simulink model "vision_try3_work"  (R2016b)
settings: Solver=VariableStepAuto  StartTime=0.0  StopTime=inf  RelTol=1e-3
undefined symbols (not defined in the file): gray
libraries: dspvision x1, visionsources x1, visionanalysis x1
settings Model: Creator=bhawnath.tiwari  LastModifiedBy=bhawnath.tiwari

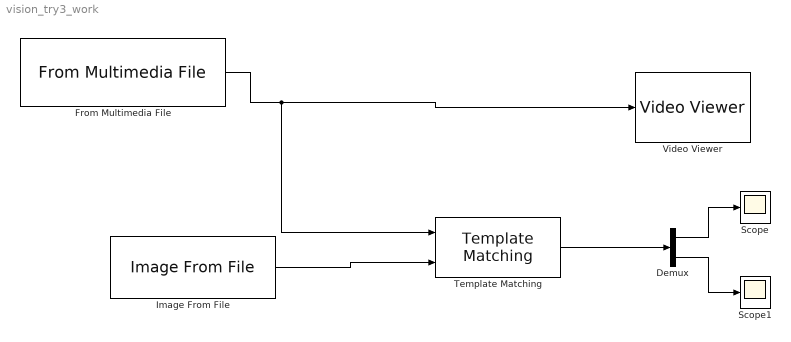
== system vision_try3_work ==
  Demux : Demux  Outputs=2
  From Multimedia File : dspvision/From Multimedia File  inputFilename=G:\Utilisateurs\bhawnath.tiwari\Documents\MATLAB\testr1.avi  loop=on  numPlays=inf  outputStreams=Video only  videoDataType=double  audioDataType=int16  inheritSampleTime=on  userDefinedSampleTime=1/30  noAudioOutput=off  isIntensityVideo=off  fourcc=Intensity  colorVideoFormat=One multidimensional signal  outputEOF=off  dataOrg=Column-major  audioFrameSize=1024  computeAudioFrameSize=off  outSamplingMode=Sample based
  Image From File : visionsources/Image From File  Tag=vipblks_nd  FileName=G:\Utilisateurs\bhawnath.tiwari\Documents\MATLAB\testr1_bolt.png  imagePorts=One multidimensional signal  Ts=inf  ImageDataType=double  Signed=on  WordLength=16  sdImageDataType=uint(8)  FractionLengthMode=User-defined  FractionLength=15  OutPortLabels=R|G|B
  Scope : Scope
  Scope1 : Scope
  Template Matching : visionanalysis/Template Matching  metric=Sum of absolute differences  output=Best match location  method=Exhaustive  nMetric=off  nSize=3  roi=off  roiValid=off  accumMode=Binary point scaling  accumWordLength=32  accumFracLength=0  prodOutputMode=Binary point scaling  prodOutputWordLength=32  prodOutputFracLength=0  roundingMode=Floor  overflowMode=off
  Video Viewer : VideoViewer  colormapValue=gray(256)  FigPos=[1 1038 1908 938]
  wires:
  From Multimedia File/1 -> Template Matching/1, Video Viewer/1
  Image From File/1 -> Template Matching/2
  Template Matching/1 -> Demux/1
  Demux/1 -> Scope/1
  Demux/2 -> Scope1/1
